simulink model "s27"  (R2023a)
settings: Solver=VariableStepAuto  StartTime=0.0  StopTime=1000.0  RelTol=1e-3
values from neighbouring files (symbols this model uses):
  A = [0 3 1 ... (first row only)    [Q1.m]    (also in Q3.m = [-2 0; SLide27.m = [2 3; 0 5 ])
  B = [10; 0; 0]    [Q1.m]    (also in Q3.m = [2; 1]; SLide27.m = [1; 2])
  C = [1 0 0]    [Q1.m]    (also in Q3.m = [3 0]; SLide27.m = [1 0)
  K = place (A,B,desrired_eignvalues2)    [Q3.m]    (also in SLide27.m = place(A,B,desiredegn))
settings Model: Creator=aalia  LastModifiedBy=aalia

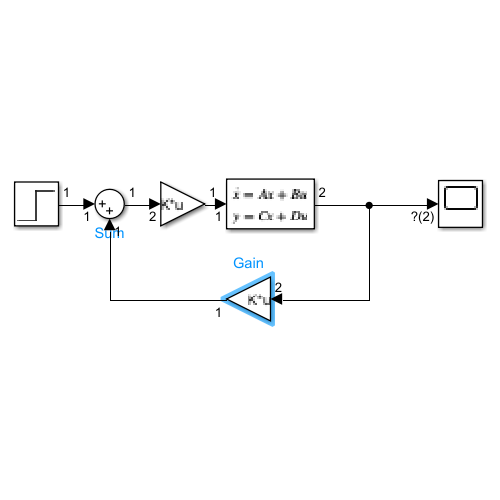
[thumbnail: Simulink's stored preview of the top-level diagram]
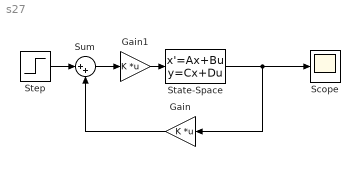
== system s27 ==
  Gain : Gain  Gain=K  Multiplication=Matrix(K*u)
  Gain1 : Gain  Gain=K  Multiplication=Matrix(K*u)
  Scope : Scope
  State-Space : StateSpace  A=A  B=B  C=C  D=[0; 0]  InitialCondition=0
  Step : Step  SampleTime=0
  Sum : Sum  Inputs=|++
  wires:
  State-Space/1 -> Gain/1, Scope/1
  Step/1 -> Sum/1
  Gain/1 -> Sum/2
  Sum/1 -> Gain1/1
  Gain1/1 -> State-Space/1
